simulink model "old_actuator_control_block"  (R2014a)
settings: Solver=ode45  StartTime=0.0  StopTime=10.0  RelTol=1e-3
undefined symbols (not defined in the file or in its folder): A1_notch_f1, A2_notch_f1, A_lpf_accel, A_lpf_dtau, B1_lpf_accel, B1_lpf_dtau, B1_notch_f1, B2_lpf_accel, B2_lpf_dtau, B2_notch_f1, j_segments, k_ff, K_notch_f1, k_sea, kd_sea_torque_flight, kd_sea_torque_stance, kp_sea_torque_flight, kp_sea_torque_stance, lateral_torque_ramp_time, max_sagittal_loaded_torque, max_sagittal_unloaded_torque, sagittal_torque_ramp_time, sample_time, sea_control_torque_cmd_small_threshold, sea_extra_moving_friction, sea_friction_sign_crossing_slope, sea_offset_friction, sea_static_friction, stance_flight_torque_threshold
libraries: simulink x7
settings Model: Creator=wmartin  LastModifiedBy=wmartin

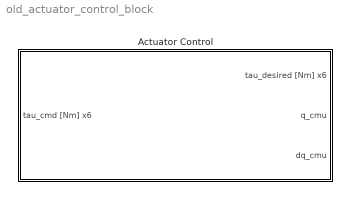
== system old_actuator_control_block ==
  Actuator Control : Subsystem

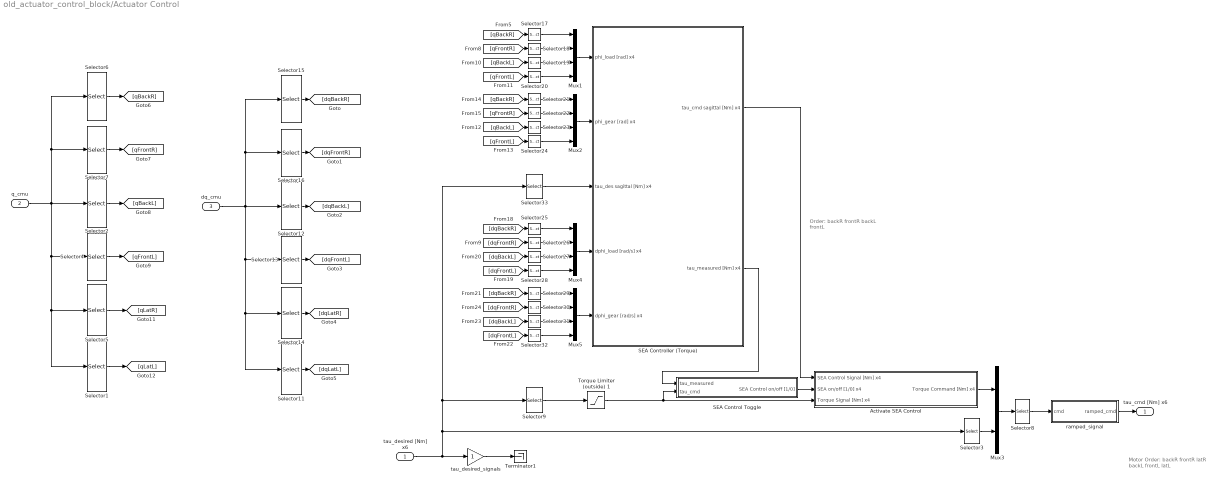
== system old_actuator_control_block/Actuator Control ==
  note: Motor Order:
      |
      | backR
      | frontR
      | latR
      | backL
      | frontL
      | latL
  note: Order:
      | backR
      | frontR
      | backL
      | frontL
  tau_desired [Nm] x6 : Inport
  q_cmu : Inport  Port=2
  dq_cmu : Inport  Port=3
  Activate SEA Control : Subsystem
  Mux{1..2,4..5} (4 alike) : Mux
  Mux3 : Mux  Inputs=2
  SEA Control Toggle : Subsystem
  SEA Controller (Torque) : Subsystem
  Selector1 : Selector  InputPortWidth=13  Indices=[10]
  Selector11 : Selector  InputPortWidth=13  Indices=[10]
  Selector12 : Selector  InputPortWidth=13  Indices=[5 6]
  Selector13 : Selector  InputPortWidth=13  Indices=[7 8]
  Selector14 : Selector  InputPortWidth=13  Indices=[9]
  Selector15 : Selector  InputPortWidth=13  Indices=[1 2]
  Selector16 : Selector  InputPortWidth=13  Indices=[3 4]
  Selector{17..20,25..28} (8 alike) : Selector  InputPortWidth=2  Indices=[1]
  Selector2 : Selector  InputPortWidth=13  Indices=[5 6]
  Selector{21..24,29..32} (8 alike) : Selector  InputPortWidth=2  Indices=[2]
  Selector3 : Selector  InputPortWidth=6  Indices=[3 6]
  Selector33 : Selector  InputPortWidth=6  Indices=[1 2 4 5]
  Selector4 : Selector  InputPortWidth=13  Indices=[7 8]
  Selector5 : Selector  InputPortWidth=13  Indices=[9]
  Selector6 : Selector  InputPortWidth=13  Indices=[1 2]
  Selector7 : Selector  InputPortWidth=13  Indices=[3 4]
  Selector8 : Selector  InputPortWidth=6  Indices=[1 2 5 3 4 6]
  Selector9 : Selector  InputPortWidth=6  Indices=[1 2 4 5]
  Terminator1 : Terminator
  Torque Limiter (outside) 1 : Saturate  UpperLimit=max_sagittal_unloaded_torque  LowerLimit=-max_sagittal_unloaded_torque
      settings: AttributesFormatString=Hi: %<UpperLimit>\nLo: %<LowerLimit>
  ramped_signal : Subsystem
  tau_desired_signals : Gain  Description=xPCTag(1)=tau_cmd_signal;
  tau_cmd [Nm] x6 : Outport  InitialOutput=[0 0 0 0 0 0]
  wires:
  Mux3/1 -> Selector8/1
  Selector3/1 -> Mux3/2
  Selector33/1 -> SEA Controller (Torque)/3(tau_des sagittal [Nm] x4)
  [dqFrontL] -> Selector32/1
  [dqBackL] -> Selector31/1
  [dqFrontR] -> Selector30/1
  Selector32/1 -> Mux5/4
  Selector30/1 -> Mux5/2
  Selector31/1 -> Mux5/3
  Selector29/1 -> Mux5/1
  [dqBackR] -> Selector29/1
  Mux5/1 -> SEA Controller (Torque)/5(dphi_gear [rad/s] x4)
  [dqFrontL] -> Selector28/1
  [dqBackL] -> Selector27/1
  [dqFrontR] -> Selector26/1
  Selector28/1 -> Mux4/4
  Selector26/1 -> Mux4/2
  Selector27/1 -> Mux4/3
  Selector25/1 -> Mux4/1
  [dqBackR] -> Selector25/1
  Mux4/1 -> SEA Controller (Torque)/4(dphi_load [rad/s] x4)
  [qFrontL] -> Selector24/1
  [qBackL] -> Selector23/1
  [qFrontR] -> Selector22/1
  Selector24/1 -> Mux2/4
  Selector22/1 -> Mux2/2
  Selector23/1 -> Mux2/3
  Selector21/1 -> Mux2/1
  [qBackR] -> Selector21/1
  Mux2/1 -> SEA Controller (Torque)/2(phi_gear [rad] x4)
  [qFrontL] -> Selector20/1
  [qBackL] -> Selector19/1
  [qFrontR] -> Selector18/1
  Selector20/1 -> Mux1/4
  Selector18/1 -> Mux1/2
  Selector19/1 -> Mux1/3
  Selector17/1 -> Mux1/1
  [qBackR] -> Selector17/1
  Mux1/1 -> SEA Controller (Torque)/1(phi_load [rad] x4)
  Selector13/1 -> [dqFrontL]
  Selector12/1 -> [dqBackL]
  Selector16/1 -> [dqFrontR]
  Selector15/1 -> [dqBackR]
  Selector11/1 -> [dqLatL]
  Selector14/1 -> [dqLatR]
  dq_cmu/1 -> Selector11/1, Selector14/1, Selector13/1, Selector15/1, Selector16/1, Selector12/1
  Selector8/1 -> ramped_signal/1(cmd)
  q_cmu/1 -> Selector2/1, Selector7/1, Selector6/1, Selector4/1, Selector5/1, Selector1/1
  Selector4/1 -> [qFrontL]
  Selector2/1 -> [qBackL]
  Selector7/1 -> [qFrontR]
  Selector6/1 -> [qBackR]
  Selector1/1 -> [qLatL]
  Selector5/1 -> [qLatR]
  tau_desired_signals/1 -> Terminator1/1
  ramped_signal/1(ramped_cmd) -> tau_cmd [Nm] x6/1
  tau_desired [Nm] x6/1 -> Selector33/1, Selector9/1, Selector3/1, tau_desired_signals/1
  Activate SEA Control/1(Torque Command [Nm] x4) -> Mux3/1
  Torque Limiter (outside) 1/1 -> Activate SEA Control/3(Torque Signal [Nm] x4), SEA Control Toggle/2(tau_cmd)
  SEA Controller (Torque)/1(tau_cmd sagittal [Nm] x4) -> Activate SEA Control/1(SEA Control Signal [Nm] x4)
  SEA Control Toggle/1(SEA Control on/off [1/0]) -> Activate SEA Control/2("SEA on/off [1/0] x4 ")
  SEA Controller (Torque)/2(tau_measured [Nm] x4) -> SEA Control Toggle/1(tau_measured)
  Selector9/1 -> Torque Limiter (outside) 1/1

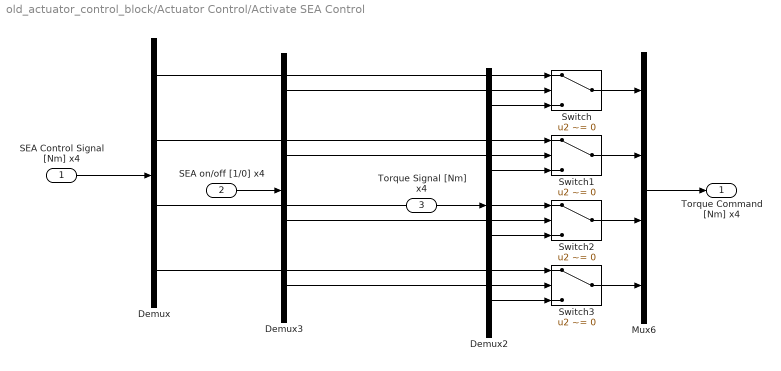
== system old_actuator_control_block/Actuator Control/Activate SEA Control ==
  SEA Control Signal [Nm] x4 : Inport
  "SEA on/off [1/0] x4 " : Inport  Port=2
  Torque Signal [Nm] x4 : Inport  Port=3
  Demux : Demux
  Demux2 : Demux
  Demux3 : Demux
  Mux6 : Mux
  Switch{,1..3} (4 alike) : Switch  Criteria=u2 ~= 0
  Torque Command [Nm] x4 : Outport
  wires:
  Demux2/2 -> Switch1/3
  Demux2/1 -> Switch/3
  Demux/1 -> Switch/1
  Switch/1 -> Mux6/1
  Switch1/1 -> Mux6/2
  Switch3/1 -> Mux6/4
  Demux3/1 -> Switch/2
  Mux6/1 -> Torque Command [Nm] x4/1
  Demux3/3 -> Switch2/2
  Demux3/2 -> Switch1/2
  Demux/3 -> Switch2/1
  Switch2/1 -> Mux6/3
  Demux/4 -> Switch3/1
  Demux2/4 -> Switch3/3
  Demux3/4 -> Switch3/2
  Demux/2 -> Switch1/1
  Demux2/3 -> Switch2/3
  SEA Control Signal [Nm] x4/1 -> Demux/1
  "SEA on/off [1/0] x4 "/1 -> Demux3/1
  Torque Signal [Nm] x4/1 -> Demux2/1

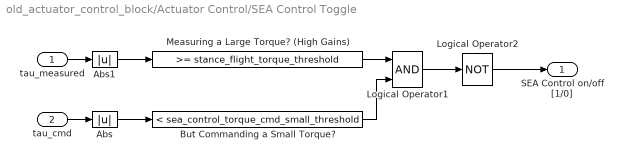
== system old_actuator_control_block/Actuator Control/SEA Control Toggle ==
  tau_measured : Inport
  tau_cmd : Inport  Port=2
  Abs : Abs
  Abs1 : Abs
  But Commanding a Small Torque? : simulink/Logic and Bit Operations/Compare To Constant  relop=<  const=sea_control_torque_cmd_small_threshold  OutDataTypeStr=boolean
  Logical Operator1 : Logic  AllPortsSameDT=off  OutDataTypeStr=boolean
  Logical Operator2 : Logic  Operator=NOT  AllPortsSameDT=off  OutDataTypeStr=boolean
  Measuring a Large Torque? (High Gains) : simulink/Logic and Bit Operations/Compare To Constant  relop=>=  const=stance_flight_torque_threshold  OutDataTypeStr=boolean
  SEA Control on/off [1/0] : Outport
  wires:
  Logical Operator2/1 -> SEA Control on/off [1/0]/1
  But Commanding a Small Torque?/1 -> Logical Operator1/2
  Logical Operator1/1 -> Logical Operator2/1
  tau_cmd/1 -> Abs/1
  Abs/1 -> But Commanding a Small Torque?/1
  tau_measured/1 -> Abs1/1
  Measuring a Large Torque? (High Gains)/1 -> Logical Operator1/1
  Abs1/1 -> Measuring a Large Torque? (High Gains)/1

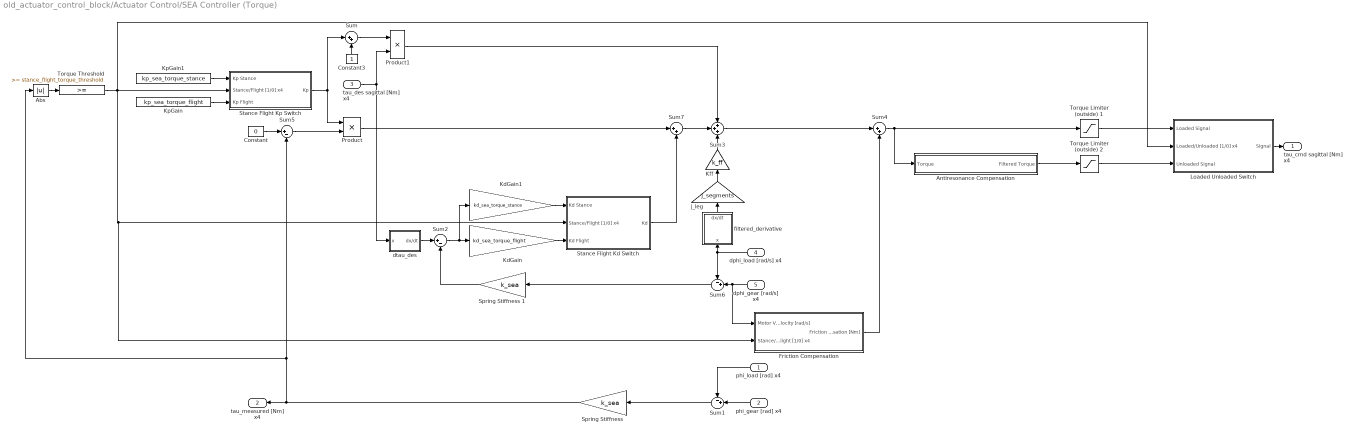
== system old_actuator_control_block/Actuator Control/SEA Controller (Torque) ==
  phi_load [rad] x4 : Inport
  phi_gear [rad] x4 : Inport  Port=2
  tau_des sagittal [Nm] x4 : Inport  Port=3
  dphi_load [rad/s] x4 : Inport  Port=4
  dphi_gear [rad/s] x4 : Inport  Port=5
  Abs : Abs
  Antiresonance Compensation : Subsystem
  Constant : Constant  Value=0
  Constant3 : Constant
  Friction Compensation : Subsystem
  KdGain : Gain  Description=xPCTag(1)=kd_sea_torque;  Gain=kd_sea_torque_flight
  KdGain1 : Gain  Description=xPCTag(1)=kd_sea_torque;  Gain=kd_sea_torque_stance
  Kff : Gain  Gain=k_ff
  KpGain : Constant  Value=kp_sea_torque_flight  SampleTime=sample_time
  KpGain1 : Constant  Value=kp_sea_torque_stance  SampleTime=sample_time
  Loaded Unloaded Switch : Subsystem
  Product : Product  SampleTime=sample_time  RndMeth=Zero
  Product1 : Product  RndMeth=Zero
  Spring Stiffness : Gain  Gain=k_sea
  Spring Stiffness 1 : Gain  Gain=k_sea
  Stance Flight Kd Switch : Subsystem
  Stance Flight Kp Switch : Subsystem
  Sum : Sum  Inputs=|++  SampleTime=sample_time
  Sum1 : Sum  Inputs=-+|
  Sum2 : Sum  Inputs=|+-
  Sum3 : Sum  Inputs=+++
  Sum4 : Sum  Inputs=|++
  Sum5 : Sum  Inputs=|+-
  Sum6 : Sum  Inputs=-+|
  Sum7 : Sum  Inputs=|++
  Torque Limiter (outside) 1 : Saturate  UpperLimit=max_sagittal_loaded_torque  LowerLimit=-max_sagittal_loaded_torque
      settings: AttributesFormatString=Hi: %<UpperLimit>\nLo: %<LowerLimit>
  Torque Limiter (outside) 2 : Saturate  UpperLimit=max_sagittal_unloaded_torque  LowerLimit=-max_sagittal_unloaded_torque
      settings: AttributesFormatString=Hi: %<UpperLimit>\nLo: %<LowerLimit>
  Torque Threshold : simulink/Logic and Bit Operations/Compare To Constant  relop=>=  const=stance_flight_torque_threshold  OutDataTypeStr=boolean
  dtau_des : Subsystem
  filtered_derivative : Subsystem
  j_leg : Gain  Description=xPCTag(1)=kd_sea_torque;  Gain=j_segments
  tau_cmd sagittal [Nm] x4 : Outport
  tau_measured [Nm] x4 : Outport  Port=2
  wires:
  Antiresonance Compensation/1(Filtered Torque) -> Torque Limiter (outside) 2/1
  Sum3/1 -> Sum4/1
  Sum7/1 -> Sum3/2
  Product1/1 -> Sum3/1
  Sum4/1 -> Antiresonance Compensation/1(Torque), Torque Limiter (outside) 1/1
  Stance Flight Kd Switch/1(Kd) -> Sum7/2
  Abs/1 -> Torque Threshold/1
  Stance Flight Kp Switch/1(Kp) -> Product/1, Sum/1
  Spring Stiffness/1 -> tau_measured [Nm] x4/1, Abs/1, Sum5/2
  KdGain1/1 -> Stance Flight Kd Switch/1(Kd Stance)
  KpGain/1 -> Stance Flight Kp Switch/3(Kp Flight)
  Torque Threshold/1 -> Loaded Unloaded Switch/2(Loaded/Unloaded [1/0] x4), Stance Flight Kp Switch/2(Stance/Flight [1/0] x4), Stance Flight Kd Switch/2(Stance/Flight [1/0] x4), Friction Compensation/2(Stance/Flight [1/0] x4)
  KpGain1/1 -> Stance Flight Kp Switch/1(Kp Stance)
  Sum1/1 -> Spring Stiffness/1
  phi_load [rad] x4/1 -> Sum1/1
  phi_gear [rad] x4/1 -> Sum1/2
  Constant/1 -> Sum5/1
  dtau_des/1(dx/dt) -> Sum2/1
  Sum6/1 -> Spring Stiffness 1/1
  Spring Stiffness 1/1 -> Sum2/2
  dphi_load [rad/s] x4/1 -> Sum6/1, filtered_derivative/1(x)
  dphi_gear [rad/s] x4/1 -> Sum6/2, Friction Compensation/1(Motor Velocity [rad/s])
  Sum2/1 -> KdGain/1, KdGain1/1
  Sum5/1 -> Product/2
  Product/1 -> Sum7/1
  KdGain/1 -> Stance Flight Kd Switch/3(Kd Flight)
  Constant3/1 -> Sum/2
  Sum/1 -> Product1/1
  filtered_derivative/1(dx/dt) -> j_leg/1
  j_leg/1 -> Kff/1
  Torque Limiter (outside) 1/1 -> Loaded Unloaded Switch/1(Loaded Signal)
  Kff/1 -> Sum3/3
  tau_des sagittal [Nm] x4/1 -> dtau_des/1(x), Product1/2
  Friction Compensation/1(Friction Compensation [Nm]) -> Sum4/2
  Torque Limiter (outside) 2/1 -> Loaded Unloaded Switch/3(Unloaded Signal)
  Loaded Unloaded Switch/1(Signal) -> tau_cmd sagittal [Nm] x4/1

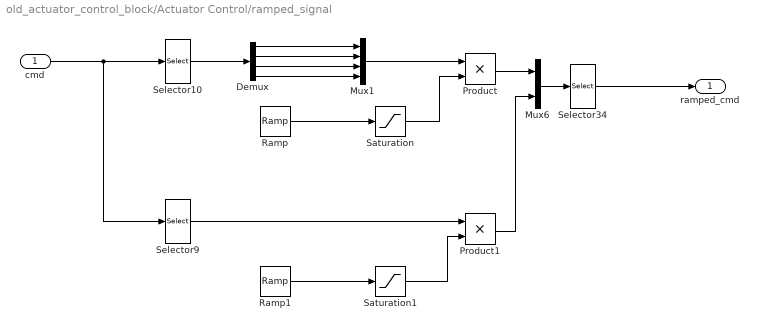
== system old_actuator_control_block/Actuator Control/ramped_signal ==
  cmd : Inport
  Demux : Demux
  Mux1 : Mux
  Mux6 : Mux  Inputs=2
  Product : Product  RndMeth=Zero
  Product1 : Product  RndMeth=Zero
  Ramp : simulink/Sources/Ramp  slope=1/sagittal_torque_ramp_time  start=sagittal_starting_time  X0=0
      settings: AttributesFormatString=Start: %<start>\nSlope: %<slope>
  Ramp1 : simulink/Sources/Ramp  slope=1/lateral_torque_ramp_time  start=control_start_time  X0=0
      settings: AttributesFormatString=Start: %<start>\nSlope: %<slope>
  Saturation : Saturate  UpperLimit=1  LowerLimit=0
      settings: AttributesFormatString=Hi: %<UpperLimit>\nLo: %<LowerLimit>
  Saturation1 : Saturate  UpperLimit=1  LowerLimit=0
      settings: AttributesFormatString=Hi: %<UpperLimit>\nLo: %<LowerLimit>
  Selector10 : Selector  InputPortWidth=6  Indices=[1 2 4 5]
  Selector34 : Selector  InputPortWidth=6  Indices=[1 2 5 3 4 6]
  Selector9 : Selector  InputPortWidth=6  Indices=[3 6]
  ramped_cmd : Outport
  wires:
  Selector9/1 -> Product1/1
  Saturation1/1 -> Product1/2
  Ramp1/1 -> Saturation1/1
  Saturation/1 -> Product/2
  Ramp/1 -> Saturation/1
  Product/1 -> Mux6/1
  cmd/1 -> Selector10/1, Selector9/1
  Product1/1 -> Mux6/2
  Selector34/1 -> ramped_cmd/1
  Selector10/1 -> Demux/1
  Mux6/1 -> Selector34/1
  Demux/1 -> Mux1/1
  Demux/2 -> Mux1/2
  Mux1/1 -> Product/1
  Demux/4 -> Mux1/4
  Demux/3 -> Mux1/3

== system old_actuator_control_block/Actuator Control/SEA Controller (Torque)/Antiresonance Compensation ==
  Torque : Inport
  Notch Filter (Flight) : DiscreteTransferFcn  Numerator=[K_notch_f1 K_notch_f1*A1_notch_f1 K_notch_f1*A2_notch_f1]  Denominator=[1 B1_notch_f1 B2_notch_f1]  SampleTime=sample_time
  Filtered Torque : Outport
  wires:
  Torque/1 -> Notch Filter (Flight)/1
  Notch Filter (Flight)/1 -> Filtered Torque/1

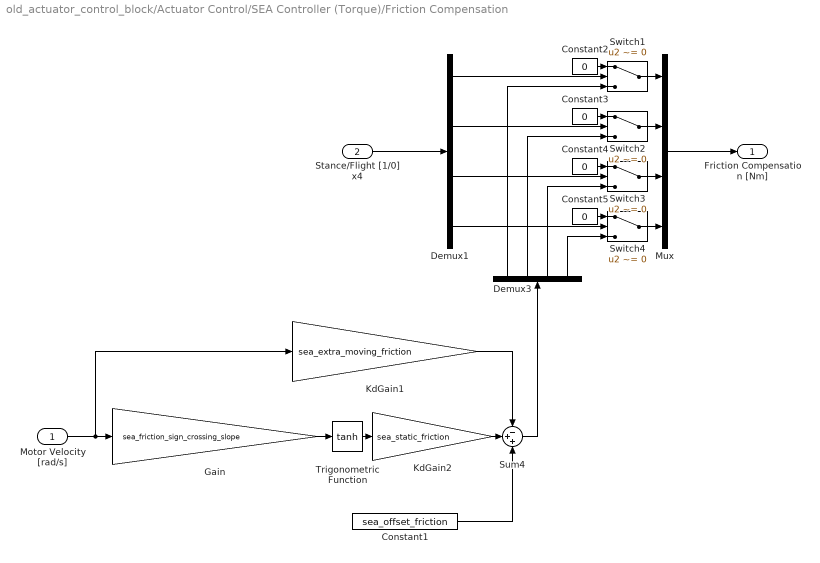
== system old_actuator_control_block/Actuator Control/SEA Controller (Torque)/Friction Compensation ==
  Motor Velocity [rad/s] : Inport
  Stance/Flight [1/0] x4 : Inport  Port=2
  Constant1 : Constant  Value=sea_offset_friction
  Constant{2..5} (4 alike) : Constant  Value=0
  Demux1 : Demux
  Demux3 : Demux
  Gain : Gain  Gain=sea_friction_sign_crossing_slope
  KdGain1 : Gain  Description=xPCTag(1)=kd_sea_torque;  Gain=sea_extra_moving_friction
  KdGain2 : Gain  Description=xPCTag(1)=kd_sea_torque;  Gain=sea_static_friction
  Mux : Mux
  Sum4 : Sum  Inputs=-++
  Switch{1..4} (4 alike) : Switch  Criteria=u2 ~= 0
  Trigonometric Function : Trigonometry  Operator=tanh
  Friction Compensation [Nm] : Outport
  wires:
  Mux/1 -> Friction Compensation [Nm]/1
  Sum4/1 -> Demux3/1
  Constant5/1 -> Switch4/1
  Constant4/1 -> Switch3/1
  Constant3/1 -> Switch2/1
  Constant2/1 -> Switch1/1
  Stance/Flight [1/0] x4/1 -> Demux1/1
  Demux3/1 -> Switch1/3
  Demux3/2 -> Switch2/3
  Demux3/3 -> Switch3/3
  Demux3/4 -> Switch4/3
  Demux1/1 -> Switch1/2
  Switch1/1 -> Mux/1
  Switch4/1 -> Mux/4
  Switch3/1 -> Mux/3
  Switch2/1 -> Mux/2
  Demux1/2 -> Switch2/2
  Demux1/3 -> Switch3/2
  Demux1/4 -> Switch4/2
  Motor Velocity [rad/s]/1 -> KdGain1/1, Gain/1
  Gain/1 -> Trigonometric Function/1
  Trigonometric Function/1 -> KdGain2/1
  KdGain2/1 -> Sum4/2
  Constant1/1 -> Sum4/3
  KdGain1/1 -> Sum4/1

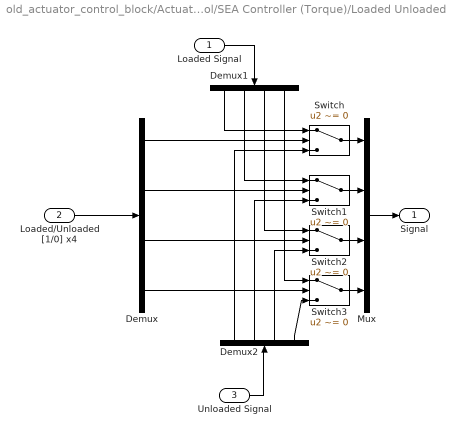
== system old_actuator_control_block/Actuator Control/SEA Controller (Torque)/Loaded Unloaded Switch ==
  Loaded Signal : Inport
  Loaded/Unloaded [1/0] x4 : Inport  Port=2
  Unloaded Signal : Inport  Port=3
  Demux : Demux
  Demux1 : Demux
  Demux2 : Demux
  Mux : Mux
  Switch{,1..3} (4 alike) : Switch  Criteria=u2 ~= 0
  Signal : Outport
  wires:
  Demux/4 -> Switch3/2
  Demux/3 -> Switch2/2
  Demux/2 -> Switch1/2
  Switch1/1 -> Mux/2
  Switch2/1 -> Mux/3
  Switch3/1 -> Mux/4
  Loaded/Unloaded [1/0] x4/1 -> Demux/1
  Mux/1 -> Signal/1
  Switch/1 -> Mux/1
  Demux/1 -> Switch/2
  Loaded Signal/1 -> Demux1/1
  Demux1/1 -> Switch/1
  Demux1/2 -> Switch1/1
  Demux1/3 -> Switch2/1
  Demux1/4 -> Switch3/1
  Unloaded Signal/1 -> Demux2/1
  Demux2/4 -> Switch3/3
  Demux2/3 -> Switch2/3
  Demux2/2 -> Switch1/3
  Demux2/1 -> Switch/3

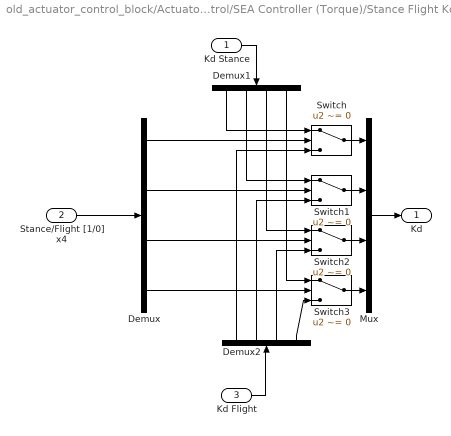
== system old_actuator_control_block/Actuator Control/SEA Controller (Torque)/Stance Flight Kd Switch ==
  Kd Stance : Inport
  Stance/Flight [1/0] x4 : Inport  Port=2
  Kd Flight : Inport  Port=3
  Demux : Demux
  Demux1 : Demux
  Demux2 : Demux
  Mux : Mux
  Switch{,1..3} (4 alike) : Switch  Criteria=u2 ~= 0
  Kd : Outport
  wires:
  Demux2/1 -> Switch/3
  Demux2/2 -> Switch1/3
  Demux2/3 -> Switch2/3
  Demux2/4 -> Switch3/3
  Kd Flight/1 -> Demux2/1
  Demux1/4 -> Switch3/1
  Demux1/3 -> Switch2/1
  Demux1/2 -> Switch1/1
  Demux1/1 -> Switch/1
  Kd Stance/1 -> Demux1/1
  Demux/1 -> Switch/2
  Switch/1 -> Mux/1
  Mux/1 -> Kd/1
  Stance/Flight [1/0] x4/1 -> Demux/1
  Switch3/1 -> Mux/4
  Switch2/1 -> Mux/3
  Switch1/1 -> Mux/2
  Demux/2 -> Switch1/2
  Demux/3 -> Switch2/2
  Demux/4 -> Switch3/2

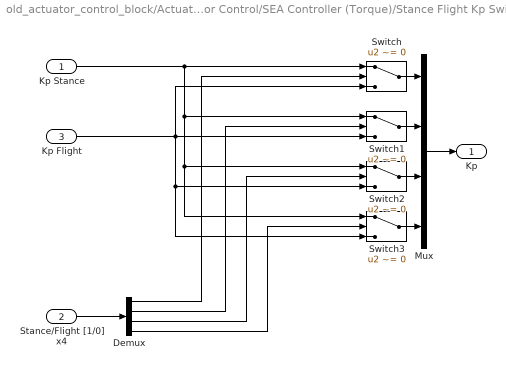
== system old_actuator_control_block/Actuator Control/SEA Controller (Torque)/Stance Flight Kp Switch ==
  Kp Stance : Inport
  Stance/Flight [1/0] x4 : Inport  Port=2
  Kp Flight : Inport  Port=3
  Demux : Demux
  Mux : Mux
  Switch{,1..3} (4 alike) : Switch  Criteria=u2 ~= 0
  Kp : Outport
  wires:
  Demux/4 -> Switch3/2
  Demux/3 -> Switch2/2
  Demux/2 -> Switch1/2
  Switch1/1 -> Mux/2
  Switch2/1 -> Mux/3
  Switch3/1 -> Mux/4
  Stance/Flight [1/0] x4/1 -> Demux/1
  Mux/1 -> Kp/1
  Switch/1 -> Mux/1
  Demux/1 -> Switch/2
  Kp Stance/1 -> Switch/1, Switch1/1, Switch2/1, Switch3/1
  Kp Flight/1 -> Switch1/3, Switch2/3, Switch3/3, Switch/3

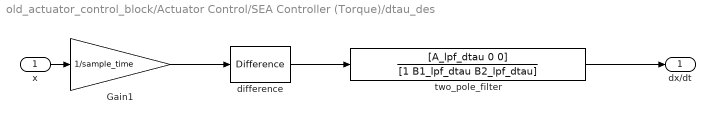
== system old_actuator_control_block/Actuator Control/SEA Controller (Torque)/dtau_des ==
  x : Inport
  Gain1 : Gain  Gain=1/sample_time
  difference : simulink/Discrete/Difference  ICPrevInput=0.0  InputProcessing=Inherited  OutMin=[]  OutMax=[]  OutDataType=fixdt(1, 16)  OutScaling=2^-10  DoSatur=off
  two_pole_filter : DiscreteTransferFcn  Numerator=[A_lpf_dtau 0 0]  Denominator=[1 B1_lpf_dtau B2_lpf_dtau]  SampleTime=sample_time
  dx/dt : Outport
  wires:
  Gain1/1 -> difference/1
  difference/1 -> two_pole_filter/1
  x/1 -> Gain1/1
  two_pole_filter/1 -> dx/dt/1

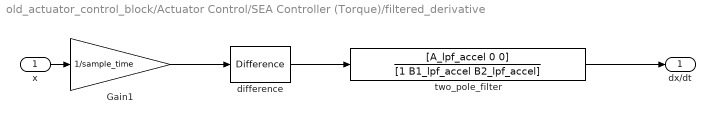
== system old_actuator_control_block/Actuator Control/SEA Controller (Torque)/filtered_derivative ==
  x : Inport
  Gain1 : Gain  Gain=1/sample_time
  difference : simulink/Discrete/Difference  ICPrevInput=0.0  InputProcessing=Inherited  OutMin=[]  OutMax=[]  OutDataType=fixdt(1, 16)  OutScaling=2^-10  DoSatur=off
  two_pole_filter : DiscreteTransferFcn  Numerator=[A_lpf_accel 0 0]  Denominator=[1 B1_lpf_accel B2_lpf_accel]  SampleTime=sample_time
  dx/dt : Outport
  wires:
  two_pole_filter/1 -> dx/dt/1
  x/1 -> Gain1/1
  difference/1 -> two_pole_filter/1
  Gain1/1 -> difference/1
